simulink model "Flowchart3"  (Simulink 6.0)
settings: Solver=FixedStepDiscrete  StartTime=0.0  StopTime=10.0  RelTol=1e-3
settings Model: Creator=scaife  LastModifiedBy=scaife  ExtModeAutoUpdateStatusClock=off

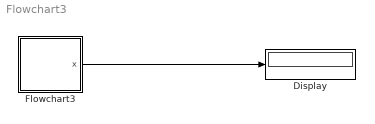
== system Flowchart3 ==
  Display : Display
  Flowchart3 : Stateflow chart
  wires:
  Flowchart3/1(x) -> Display/1

== stateflow chart Flowchart3 ==
  state A [parallel]
    A -> (junction 4) : {x++;}
  data: x output int32
